simulink model "Attenuation_freespace_propagation"  (Simulink 7.5)
settings: Solver=ode45  StartTime=0.0  StopTime=10.0  RelTol=1e-3
undefined symbols (not defined in the file): magnitude
settings Model: Creator=J HUANG  LastModifiedBy=J HUANG

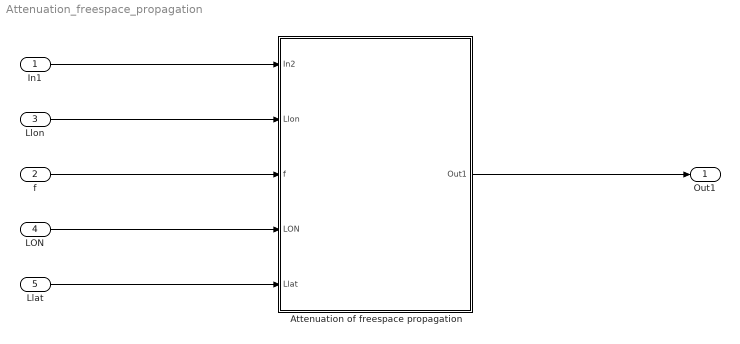
== system Attenuation_freespace_propagation ==
  In1 : Inport  OutDataType=fixdt(1, 16)  OutScaling=2^0
  f : Inport  Port=2  OutDataType=fixdt(1, 16)  OutScaling=2^0
  Llon : Inport  Port=3  OutDataType=fixdt(1, 16)  OutScaling=2^0
  LON : Inport  Port=4  OutDataType=fixdt(1, 16)  OutScaling=2^0
  Llat : Inport  Port=5  OutDataType=fixdt(1, 16)  OutScaling=2^0
  Attenuation of freespace propagation : Subsystem
  Out1 : Outport  OutDataType=fixdt(1, 16)  OutScaling=2^0
  wires:
  In1/1 -> Attenuation of freespace propagation/1(In2)
  Attenuation of freespace propagation/1(Out1) -> Out1/1
  f/1 -> Attenuation of freespace propagation/3(f)
  Llon/1 -> Attenuation of freespace propagation/2(Llon)
  LON/1 -> Attenuation of freespace propagation/4(LON)
  Llat/1 -> Attenuation of freespace propagation/5(Llat)

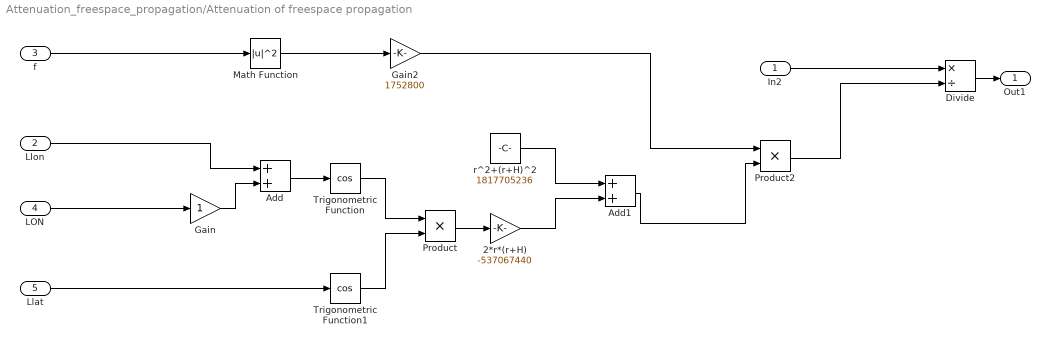
== system Attenuation_freespace_propagation/Attenuation of freespace propagation ==
  In2 : Inport
  Llon : Inport  Port=2  OutDataType=fixdt(1, 16)  OutScaling=2^0
  f : Inport  Port=3  OutDataType=fixdt(1, 16)  OutScaling=2^0
  LON : Inport  Port=4  OutDataType=fixdt(1, 16)  OutScaling=2^0
  Llat : Inport  Port=5  OutDataType=fixdt(1, 16)  OutScaling=2^0
  2*r*(r+H) : Gain  Gain=-537067440  ParameterDataType=fixdt(1, 16)  ParameterScaling=2^0  OutDataType=fixdt(1, 16)  OutScaling=2^0
  Add : Sum  OutDataType=fixdt(1, 16)  OutScaling=2^-10
  Add1 : Sum  OutDataType=fixdt(1, 16)  OutScaling=2^-10
  Divide : Product  Inputs=*/  OutDataType=fixdt(1, 16)  OutScaling=2^-10
  Gain : Gain  ParameterDataType=fixdt(1, 16)  ParameterScaling=2^0  OutDataType=fixdt(1, 16)  OutScaling=2^0
  Gain2 : Gain  Gain=1752800  ParameterDataType=fixdt(1, 16)  ParameterScaling=2^0  OutDataType=fixdt(1, 16)  OutScaling=2^0
  Math Function : Math  Operator=magnitude^2  OutDataType=fixdt(1, 16)  OutScaling=2^0  SaturateOnIntegerOverflow=on
  Product : Product  OutDataType=fixdt(1, 16)  OutScaling=2^0  RndMeth=Zero
  Product2 : Product  OutDataType=fixdt(1, 16)  OutScaling=2^0  RndMeth=Zero
  Trigonometric Function : Trigonometry  Operator=cos
  Trigonometric Function1 : Trigonometry  Operator=cos
  r^2+(r+H)^2 : Constant  Value=1817705236  OutDataType=fixdt(1, 16)  OutScaling=2^0
  Out1 : Outport
  wires:
  Llat/1 -> Trigonometric Function1/1
  Llon/1 -> Add/1
  LON/1 -> Gain/1
  f/1 -> Math Function/1
  Product2/1 -> Divide/2
  Add1/1 -> Product2/2
  Gain2/1 -> Product2/1
  Math Function/1 -> Gain2/1
  2*r*(r+H)/1 -> Add1/2
  r^2+(r+H)^2/1 -> Add1/1
  Product/1 -> 2*r*(r+H)/1
  Trigonometric Function1/1 -> Product/2
  Trigonometric Function/1 -> Product/1
  Add/1 -> Trigonometric Function/1
  Gain/1 -> Add/2
  In2/1 -> Divide/1
  Divide/1 -> Out1/1
